simulink model "Simulank_file"  (R2022b)
settings: Solver=VariableStepAuto  StartTime=0.0  StopTime=0.2  MaxStep=0.001  RelTol=1e-3
values from neighbouring files (symbols this model uses):
  C = 1    [script_file.m]
  R = 1    [script_file.m]
libraries: simulink x1
settings Model: Creator=ahmed  LastModifiedBy=ahmed

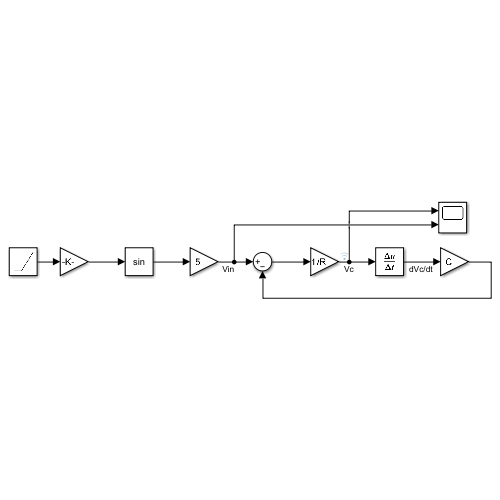
[thumbnail: Simulink's stored preview of the top-level diagram]
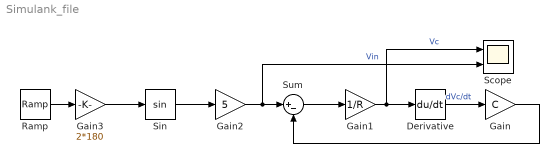
== system Simulank_file ==
  Derivative : Derivative
  Gain : Gain  Gain=C
  Gain1 : Gain  Gain=1/R
  Gain2 : Gain  Gain=5
  Gain3 : Gain  Gain=2*180
  Ramp : simulink/Sources/Ramp  slope=1  start=0  InitialOutput=0
  Scope : Scope  NumInputPorts=2
  Sin : Trigonometry
  Sum : Sum  Inputs=|+-
  wires:
  Gain/1 -> Sum/2
  Ramp/1 -> Gain3/1
  Gain3/1 -> Sin/1
  Derivative/1 -> Gain/1  "dVc/dt"
  Gain2/1 -> Scope/2, Sum/1  "Vin"
  Sin/1 -> Gain2/1
  Sum/1 -> Gain1/1
  Gain1/1 -> Scope/1, Derivative/1  "Vc"
